simulink model "byteviewer"  (Simulink 3.00)
settings: Solver=ode45  StartTime=0.0  StopTime=10.0  RelTol=1e-3
settings Model: LastModifiedBy=campa

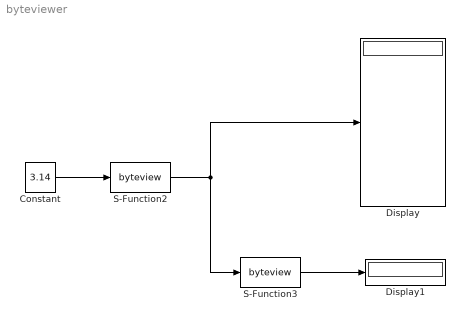
== system byteviewer ==
  Constant : Constant  Value=3.14
  Display : Display
      settings: Format=short
  Display1 : Display
      settings: Format=short
  S-Function2 : S-Function  FunctionName=byteview  Parameters=Ni,Ti,To  PortCounts=[]  SFunctionModules=''  mask(Byte Viewer){Ni=1, Ti=double, To=uint8}
      mask prompts: Ni "Number of inputs (Ni)"; Ti "Input Type (Ti)"; To "Output Type (To)"
      mask help:
      | This block takes in input a vector of Ni signals belonging to a type Ti,
      |   puts them all in a contiguous memory zone, and reinterprets them as
      |   a vector of No signals belonging to a type To.
      |   The number of outputs No is equal to Ni*sizeof(To)/sizeof(Ti),
      |   where sizeof is the number of bytes of the type.
      mask Help:
      | This block takes in input a vector of Ni signals belonging to a type Ti,
      |   puts them all in a contiguous memory zone, and reinterprets them as
      |   a vector of No signals belonging to a type To.
      |   The number of outputs No is equal to Ni*sizeof(To)/sizeof(Ti),
      |   where sizeof is the number of bytes of the type.
      | 
      |   Typically you can use this block to decompose/recompose a double
      |   or a float into/from the bytes that composes it.
      mask StyleString: edit,popup(double|single|int8|uint8|int16|uint16|int32|uint32|boolean),popup(double|single|int8|uint8|int16|uint16|int32|uint32|boolean)
  S-Function3 : S-Function  FunctionName=byteview  Parameters=Ni,Ti,To  PortCounts=[]  SFunctionModules=''  mask(Byte Viewer){Ni=8, Ti=uint8, To=double}
      mask prompts: Ni "Number of inputs (Ni)"; Ti "Input Type (Ti)"; To "Output Type (To)"
      mask help:
      | This block takes in input a vector of Ni signals belonging to a type Ti,
      |   puts them all in a contiguous memory zone, and reinterprets them as
      |   a vector of No signals belonging to a type To.
      |   The number of outputs No is equal to Ni*sizeof(To)/sizeof(Ti),
      |   where sizeof is the number of bytes of the type.
      mask Help:
      | This block takes in input a vector of Ni signals belonging to a type Ti,
      |   puts them all in a contiguous memory zone, and reinterprets them as
      |   a vector of No signals belonging to a type To.
      |   The number of outputs No is equal to Ni*sizeof(To)/sizeof(Ti),
      |   where sizeof is the number of bytes of the type.
      | 
      |   Typically you can use this block to decompose/recompose a double
      |   or a float into/from the bytes that composes it.
      mask StyleString: edit,popup(double|single|int8|uint8|int16|uint16|int32|uint32|boolean),popup(double|single|int8|uint8|int16|uint16|int32|uint32|boolean)
  wires:
  Constant/1 -> S-Function2/1
  S-Function2/1 -> Display/1, S-Function3/1
  S-Function3/1 -> Display1/1
